simulink model "sixth_harmonic_concen"  (R2013a)
settings: Solver=ode4  StartTime=0.0  StopTime=0.1  FixedStep=Ts  RelTol=1e-3
values from neighbouring files (symbols this model uses):
  Cdc = 100e-6    (= 0.0001)    [acemp_sixth.m]    (also in immd_design_elen.m = 0.0002; immd_efficiency.m = 5e-05; immd_simulation_base.m = 5e-05; sixth_harmonic_report.m = 0.003)
  injfreq = 300*2*pi    (= 1884.95559215)    [acemp_sixth.m]
  injphase = k*pi/180    [acemp_sixth.m]
  injvoltmagn = 20    [acemp_sixth.m]
  Lload = Xload/wout_fund    [acemp_sixth.m]    (also in immd_base_varyingmod.m = Xload/wout; immd_design_elen.m = Xload/wout; immd_efficiency.m = Xload/wout; immd_simulation_base.m = Xload/wout)
  ma1 = 0.8    [acemp_sixth.m]
  ma3 = 0.5    [acemp_sixth.m]
  R1 = 5    [acemp_sixth.m]    (also in immd_efficiency.m; immd_simulation_base.m)
  Rload = Zload*pf    (= 17.306929152)    [acemp_sixth.m]    (also in immd_base_varyingmod.m = Zload*pf; immd_design_elen.m = Zload*pf; immd_efficiency.m = Zload*pf; immd_simulation_base.m = Zload*pf)
  Ts = 1e-6    (= 1e-06)    [acemp_sixth.m]    (also in immd_base_varyingmod.m = 1e-05; immd_design_elen.m; immd_efficiency.m; immd_simulation_base.m)
  V1 = Vdc*(R1+Rrefl)/Rrefl    (= 475.757575758)    [acemp_sixth.m]    (also in immd_efficiency.m = 526.262626263; immd_simulation_base.m = 425.252525253)
  wout_fund = 2*pi*fout_fund    (= 314.159265359)    [acemp_sixth.m]
  wout_three = 2*pi*fout_three    (= 942.477796077)    [acemp_sixth.m]
libraries: powerlib x33, powerlib_meascontrol x28
settings Model: Creator=ugurm  LastModifiedBy=ugurm

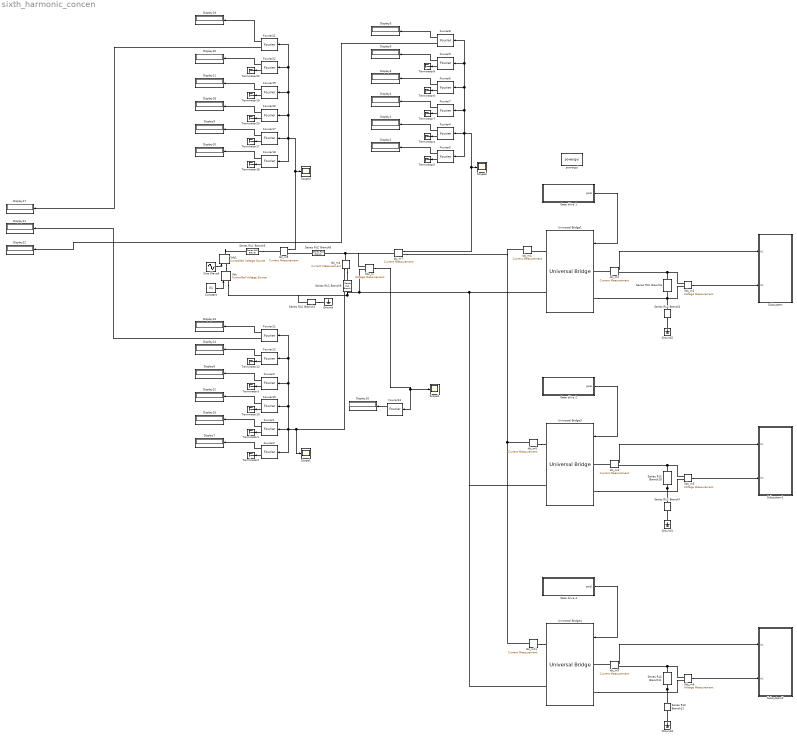
== system sixth_harmonic_concen ==
  Constant : Constant  Value=V1
  Display{1..22} (22 alike) : Display
  Fourier1 : powerlib_meascontrol/Measurements/Fourier  Freq=fout_fund  n=1  InInit=[0, 0]  Ts=Ts
  Fourier10 : powerlib_meascontrol/Measurements/Fourier  Freq=fout_fund  n=2  InInit=[0, 0]  Ts=Ts
  Fourier11 : powerlib_meascontrol/Measurements/Fourier  Freq=fout_fund  n=6  InInit=[0, 0]  Ts=Ts
  Fourier12 : powerlib_meascontrol/Measurements/Fourier  Freq=fout_fund  n=4  InInit=[0, 0]  Ts=Ts
  Fourier{2,5,13,18} (4 alike) : powerlib_meascontrol/Measurements/Fourier  Freq=fout_fund  n=0  InInit=[0, 0]  Ts=Ts
  Fourier17 : powerlib_meascontrol/Measurements/Fourier  Freq=fout_fund  n=1  InInit=[0, 0]  Ts=Ts
  Fourier19 : powerlib_meascontrol/Measurements/Fourier  Freq=fout_fund  n=3  InInit=[0, 0]  Ts=Ts
  Fourier20 : powerlib_meascontrol/Measurements/Fourier  Freq=fout_fund  n=2  InInit=[0, 0]  Ts=Ts
  Fourier21 : powerlib_meascontrol/Measurements/Fourier  Freq=fout_fund  n=6  InInit=[0, 0]  Ts=Ts
  Fourier22 : powerlib_meascontrol/Measurements/Fourier  Freq=fout_fund  n=4  InInit=[0, 0]  Ts=Ts
  Fourier3 : powerlib_meascontrol/Measurements/Fourier  Freq=fout_fund  n=3  InInit=[0, 0]  Ts=Ts
  Fourier4 : powerlib_meascontrol/Measurements/Fourier  Freq=fout_fund  n=1  InInit=[0, 0]  Ts=Ts
  Fourier6 : powerlib_meascontrol/Measurements/Fourier  Freq=fout_fund  n=3  InInit=[0, 0]  Ts=Ts
  Fourier7 : powerlib_meascontrol/Measurements/Fourier  Freq=fout_fund  n=2  InInit=[0, 0]  Ts=Ts
  Fourier8 : powerlib_meascontrol/Measurements/Fourier  Freq=fout_fund  n=6  InInit=[0, 0]  Ts=Ts
  Fourier9 : powerlib_meascontrol/Measurements/Fourier  Freq=fout_fund  n=4  InInit=[0, 0]  Ts=Ts
  Gate drive 1 : Subsystem
  Gate drive 2 : Subsystem
  Gate drive 4 : Subsystem
  Ground{,1..3} (4 alike) : powerlib/Elements/Ground  LConnTagsString=a
  Idc_m{1..7,9,11} (9 alike) : powerlib/Measurements/Current Measurement  PhasorSimulation=off  OutputType=Complex  PSBequivalent=0
  Scope{1..4} (4 alike) : Scope
      Scope1 settings: TimeRange=0.05  YMin=-15  YMax=42.5  SaveName=idc2
      Scope2 settings: TimeRange=0.05  YMin=380  YMax=422.5  SaveName=idc3
      Scope3 settings: TimeRange=0.05  YMin=-17.5  YMax=32.5  SaveName=idc
      Scope4 settings: TimeRange=0.05  YMin=10  YMax=25  SaveName=idc1
  Series RLC Branch10 : powerlib/Elements/Series RLC Branch  LConnTagsString=__new0  RConnTagsString=__new0  BranchType=RL  Resistance=Rload  Inductance=Lload  SetiL0=off  InitialCurrent=0  Capacitance=1e-6  Setx0=off  InitialVoltage=0  Measurements=None
  Series RLC Branch11 : powerlib/Elements/Series RLC Branch  LConnTagsString=__new0  RConnTagsString=__new0  BranchType=RL  Resistance=Rload  Inductance=Lload  SetiL0=off  InitialCurrent=0  Capacitance=1e-6  Setx0=off  InitialVoltage=0  Measurements=None
  Series RLC Branch{2..3,7,12} (4 alike) : powerlib/Elements/Series RLC Branch  LConnTagsString=__new0  RConnTagsString=__new0  BranchType=R  Resistance=1e12  Inductance=Lload  SetiL0=off  InitialCurrent=0  Capacitance=1e-6  Setx0=off  InitialVoltage=0  Measurements=None
  Series RLC Branch5 : powerlib/Elements/Series RLC Branch  LConnTagsString=__new0  RConnTagsString=__new0  BranchType=L  Resistance=1  Inductance=1e-3  SetiL0=off  InitialCurrent=0  Capacitance=1e-6  Setx0=off  InitialVoltage=0  Measurements=None
  Series RLC Branch6 : powerlib/Elements/Series RLC Branch  LConnTagsString=__new0  RConnTagsString=__new0  BranchType=RL  Resistance=Rload  Inductance=Lload  SetiL0=off  InitialCurrent=0  Capacitance=1e-6  Setx0=off  InitialVoltage=0  Measurements=None
  Series RLC Branch8 : powerlib/Elements/Series RLC Branch  LConnTagsString=__new0  RConnTagsString=__new0  BranchType=R  Resistance=R1  Inductance=Lload  SetiL0=off  InitialCurrent=0  Capacitance=1e-6  Setx0=off  InitialVoltage=0  Measurements=None
  Series RLC Branch9 : powerlib/Elements/Series RLC Branch  LConnTagsString=__new0  RConnTagsString=__new0  BranchType=C  Resistance=1e12  Inductance=Lload  SetiL0=off  InitialCurrent=0  Capacitance=Cdc  Setx0=off  InitialVoltage=0  Measurements=None
  Sine Wave3 : Sin  Amplitude=injvoltmagn  Frequency=injfreq  Phase=injphase  SampleTime=0
  Subsystem : Subsystem
  Subsystem1 : Subsystem
  Subsystem2 : Subsystem
  Terminator{1..7,9..10,12,17..20,22} (15 alike) : Terminator
  Universal Bridge1 : powerlib/Power Electronics/Universal Bridge  Arms=2  SnubberResistance=1e5  SnubberCapacitance=inf  Device=IGBT / Diodes  Ron=1e-6  Lon=0  ForwardVoltages="[  0  0  ]"  ForwardVoltage=0  GTOparameters=[ 10e-6 , 20e-6 ]  IGBTparameters=[0,0]  Measurements=None  Measurements_2=None  converterType=Rectifier
  Universal Bridge3 : powerlib/Power Electronics/Universal Bridge  Arms=2  SnubberResistance=1e5  SnubberCapacitance=inf  Device=IGBT / Diodes  Ron=1e-6  Lon=0  ForwardVoltages="[  0  0  ]"  ForwardVoltage=0  GTOparameters=[ 10e-6 , 20e-6 ]  IGBTparameters=[0,0]  Measurements=None  Measurements_2=None  converterType=Rectifier
  Universal Bridge4 : powerlib/Power Electronics/Universal Bridge  Arms=2  SnubberResistance=1e5  SnubberCapacitance=inf  Device=IGBT / Diodes  Ron=1e-6  Lon=0  ForwardVoltages="[  0  0  ]"  ForwardVoltage=0  GTOparameters=[ 10e-6 , 20e-6 ]  IGBTparameters=[0,0]  Measurements=None  Measurements_2=None  converterType=Rectifier
  Vdc : powerlib/Electrical Sources/Controlled Voltage Source  Initialize=off  Source_Type=DC  Amplitude=200  Phase=0  Frequency=0  Measurements=None
  Vdc1 : powerlib/Electrical Sources/Controlled Voltage Source  Initialize=off  Source_Type=DC  Amplitude=200  Phase=0  Frequency=0  Measurements=None
  Vdc_m{,2,5..6} (4 alike) : powerlib/Measurements/Voltage Measurement  PhasorSimulation=off  OutputType=Complex  PSBequivalent=0
  powergui : powerlib/powergui  Priority=1  SimulationMode=Discrete  SolverType=Tustin  SampleTime=Ts  frequency=60  SPID=off  DisableSnubberDevices=off  DisableRonSwitches=off  DisableVfSwitches=off  SwTol=0  Interpol=off  DisplayEquations=off  frequencyindice=0  Pbase=100e6  ErrMax=1e-4  Iterations=50  UnitsV=kV  UnitsW=MW  FunctionMessages=off  echomessages=off  HookPort=off  EnableUseOfTLC=off  x0status=blocks  RestoreLinks=warning  ResistiveCurrentMeasurement=off  Frange=[0:2:500]  Ylog=off  Xlog=on  ShowGrid=off  save=off  variable=ZData  structure=idc2  ZoomFFT=off  StartTime=0.02  cycles=4  DisplayStyle=2  fundamental=50  FreqAxis=off  MaxFrequency=1000  frequencyindicesteady=1  RmsSteady=1  display=off  Ts=0  methode=off
  wires:
  Gate drive 1/1(gate1) -> Universal Bridge1/1
  Fourier4/1 -> Display1/1
  Fourier4/2 -> Terminator4/1
  Fourier5/1 -> Display2/1
  Fourier5/2 -> Terminator5/1
  Fourier6/1 -> Display3/1
  Fourier6/2 -> Terminator6/1
  Fourier7/1 -> Display4/1
  Fourier7/2 -> Terminator7/1
  Fourier8/1 -> Display5/1
  Fourier8/2 -> Display22/1
  Idc_m7/1 -> Scope3/1, Fourier8/1, Fourier9/1, Fourier6/1, Fourier7/1, Fourier5/1, Fourier4/1
  Fourier9/1 -> Display6/1
  Fourier9/2 -> Terminator9/1
  Idc_m2/1 -> Subsystem/1(In1)
  Vdc_m2/1 -> Subsystem/2(In2)
  Gate drive 2/1(gate1) -> Universal Bridge3/1
  Idc_m3/1 -> Subsystem1/1(In1)
  Vdc_m5/1 -> Subsystem1/2(In2)
  Fourier17/1 -> Display9/1
  Fourier17/2 -> Terminator17/1
  Fourier18/1 -> Display10/1
  Fourier18/2 -> Terminator18/1
  Fourier19/1 -> Display11/1
  Fourier19/2 -> Terminator19/1
  Fourier20/1 -> Display18/1
  Fourier20/2 -> Terminator20/1
  Fourier21/1 -> Display19/1
  Fourier21/2 -> Display17/1
  Idc_m5/1 -> Scope4/1, Fourier21/1, Fourier22/1, Fourier19/1, Fourier20/1, Fourier18/1, Fourier17/1
  Fourier22/1 -> Display20/1
  Fourier22/2 -> Terminator22/1
  Gate drive 4/1(gate1) -> Universal Bridge4/1
  Idc_m9/1 -> Subsystem2/1(In1)
  Vdc_m6/1 -> Subsystem2/2(In2)
  Constant/1 -> Vdc/1
  Sine Wave3/1 -> Vdc1/1
  Fourier1/1 -> Display15/1
  Fourier1/2 -> Terminator1/1
  Fourier2/1 -> Display7/1
  Fourier2/2 -> Terminator2/1
  Fourier3/1 -> Display8/1
  Fourier3/2 -> Terminator3/1
  Fourier10/1 -> Display12/1
  Fourier10/2 -> Terminator10/1
  Fourier11/1 -> Display13/1
  Fourier11/2 -> Display21/1
  Idc_m4/1 -> Scope1/1, Fourier11/1, Fourier12/1, Fourier3/1, Fourier10/1, Fourier2/1, Fourier1/1
  Fourier12/1 -> Display14/1
  Fourier12/2 -> Terminator12/1
  Vdc_m/1 -> Fourier13/1, Scope2/1
  Fourier13/1 -> Display16/1
  connections:
  Universal Bridge1/RConn1 -- Idc_m1/RConn1
  Universal Bridge1/LConn2 -- Series RLC Branch2/LConn1 -- Vdc_m2/LConn2 -- Series RLC Branch6/RConn1
  Idc_m2/LConn1 -- Universal Bridge1/LConn1
  Series RLC Branch6/LConn1 -- Vdc_m2/LConn1 -- Idc_m2/RConn1
  Ground2/LConn1 -- Series RLC Branch2/RConn1
  Series RLC Branch9/RConn1 -- Vdc_m/LConn2 -- Universal Bridge1/RConn2 -- Universal Bridge4/RConn2 -- Universal Bridge3/RConn2 -- Vdc/LConn1 -- Series RLC Branch3/LConn1
  Idc_m4/LConn1 -- Vdc_m/LConn1 -- Idc_m7/LConn1 -- Series RLC Branch8/LConn1
  Series RLC Branch10/RConn1 -- Series RLC Branch7/LConn1 -- Universal Bridge3/LConn2 -- Vdc_m5/LConn2
  Series RLC Branch10/LConn1 -- Vdc_m5/LConn1 -- Idc_m3/RConn1
  Ground1/LConn1 -- Series RLC Branch7/RConn1
  Idc_m3/LConn1 -- Universal Bridge3/LConn1
  Idc_m6/RConn1 -- Universal Bridge3/RConn1
  Series RLC Branch11/RConn1 -- Series RLC Branch12/LConn1 -- Universal Bridge4/LConn2 -- Vdc_m6/LConn2
  Series RLC Branch11/LConn1 -- Vdc_m6/LConn1 -- Idc_m9/RConn1
  Ground3/LConn1 -- Series RLC Branch12/RConn1
  Idc_m9/LConn1 -- Universal Bridge4/LConn1
  Idc_m11/RConn1 -- Universal Bridge4/RConn1
  Series RLC Branch3/RConn1 -- Ground/LConn1
  Series RLC Branch8/RConn1 -- Idc_m5/RConn1
  Series RLC Branch5/LConn1 -- Idc_m5/LConn1
  Idc_m4/RConn1 -- Series RLC Branch9/LConn1
  Vdc1/RConn1 -- Series RLC Branch5/RConn1
  Vdc1/LConn1 -- Vdc/RConn1
  Idc_m11/LConn1 -- Idc_m1/LConn1 -- Idc_m7/RConn1 -- Idc_m6/LConn1

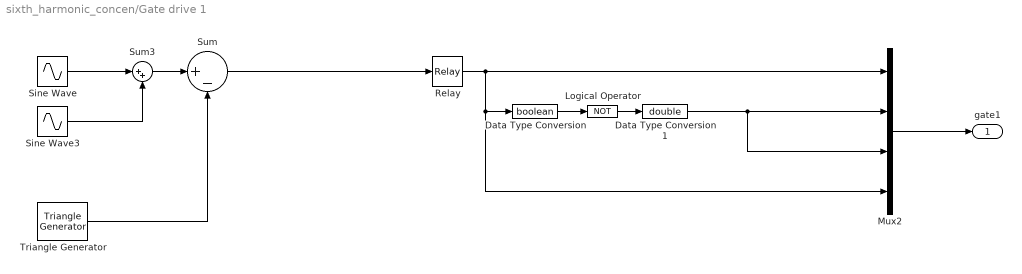
== system sixth_harmonic_concen/Gate drive 1 ==
  Data Type Conversion : DataTypeConversion  OutDataTypeStr=boolean
  Data Type Conversion1 : DataTypeConversion  OutDataTypeStr=double
  Logical Operator : Logic  Operator=NOT  AllPortsSameDT=off  OutDataTypeStr=boolean
  Mux2 : Mux
  Relay : Relay
  Sine Wave : Sin  Amplitude=ma1  Frequency=wout_fund  SampleTime=0
  Sine Wave3 : Sin  Amplitude=ma3  Frequency=wout_three  SampleTime=0
  Sum : Sum  Inputs=|+-
  Sum3 : Sum  Inputs=|++
  Triangle Generator : powerlib_meascontrol/Pulse & Signal Generators/Triangle Generator  Freq=fsw  Phase=0  Ts=Ts
  gate1 : Outport
  wires:
  Sum/1 -> Relay/1
  Data Type Conversion/1 -> Logical Operator/1
  Relay/1 -> Mux2/4, Data Type Conversion/1, Mux2/1
  Logical Operator/1 -> Data Type Conversion1/1
  Data Type Conversion1/1 -> Mux2/2, Mux2/3
  Mux2/1 -> gate1/1
  Sine Wave/1 -> Sum3/1
  Sine Wave3/1 -> Sum3/2
  Sum3/1 -> Sum/1
  Triangle Generator/1 -> Sum/2

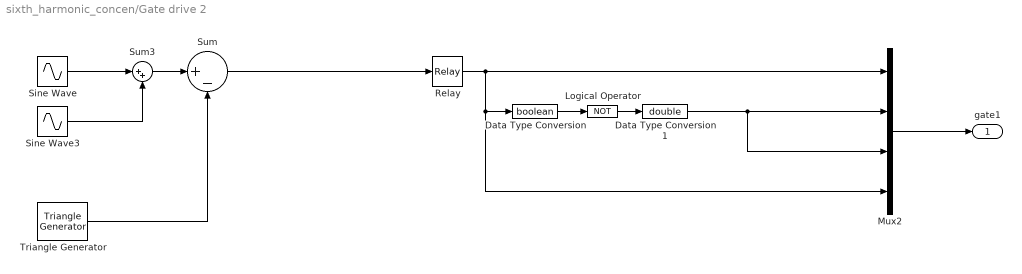
== system sixth_harmonic_concen/Gate drive 2 ==
  Data Type Conversion : DataTypeConversion  OutDataTypeStr=boolean
  Data Type Conversion1 : DataTypeConversion  OutDataTypeStr=double
  Logical Operator : Logic  Operator=NOT  AllPortsSameDT=off  OutDataTypeStr=boolean
  Mux2 : Mux
  Relay : Relay
  Sine Wave : Sin  Amplitude=ma1  Frequency=wout_fund  Phase=-2*pi/3  SampleTime=0
  Sine Wave3 : Sin  Amplitude=ma3  Frequency=wout_three  SampleTime=0
  Sum : Sum  Inputs=|+-
  Sum3 : Sum  Inputs=|++
  Triangle Generator : powerlib_meascontrol/Pulse & Signal Generators/Triangle Generator  Freq=fsw  Phase=0  Ts=Ts
  gate1 : Outport
  wires:
  Sum/1 -> Relay/1
  Data Type Conversion/1 -> Logical Operator/1
  Relay/1 -> Mux2/4, Data Type Conversion/1, Mux2/1
  Logical Operator/1 -> Data Type Conversion1/1
  Data Type Conversion1/1 -> Mux2/2, Mux2/3
  Mux2/1 -> gate1/1
  Sine Wave/1 -> Sum3/1
  Sine Wave3/1 -> Sum3/2
  Sum3/1 -> Sum/1
  Triangle Generator/1 -> Sum/2

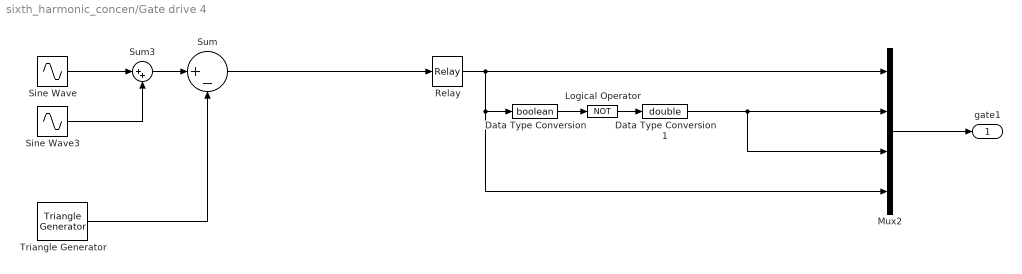
== system sixth_harmonic_concen/Gate drive 4 ==
  Data Type Conversion : DataTypeConversion  OutDataTypeStr=boolean
  Data Type Conversion1 : DataTypeConversion  OutDataTypeStr=double
  Logical Operator : Logic  Operator=NOT  AllPortsSameDT=off  OutDataTypeStr=boolean
  Mux2 : Mux
  Relay : Relay
  Sine Wave : Sin  Amplitude=ma1  Frequency=wout_fund  Phase=-4*pi/3  SampleTime=0
  Sine Wave3 : Sin  Amplitude=ma3  Frequency=wout_three  SampleTime=0
  Sum : Sum  Inputs=|+-
  Sum3 : Sum  Inputs=|++
  Triangle Generator : powerlib_meascontrol/Pulse & Signal Generators/Triangle Generator  Freq=fsw  Phase=0  Ts=Ts
  gate1 : Outport
  wires:
  Sum/1 -> Relay/1
  Data Type Conversion/1 -> Logical Operator/1
  Relay/1 -> Mux2/4, Data Type Conversion/1, Mux2/1
  Logical Operator/1 -> Data Type Conversion1/1
  Data Type Conversion1/1 -> Mux2/2, Mux2/3
  Mux2/1 -> gate1/1
  Sine Wave/1 -> Sum3/1
  Sine Wave3/1 -> Sum3/2
  Sum3/1 -> Sum/1
  Triangle Generator/1 -> Sum/2

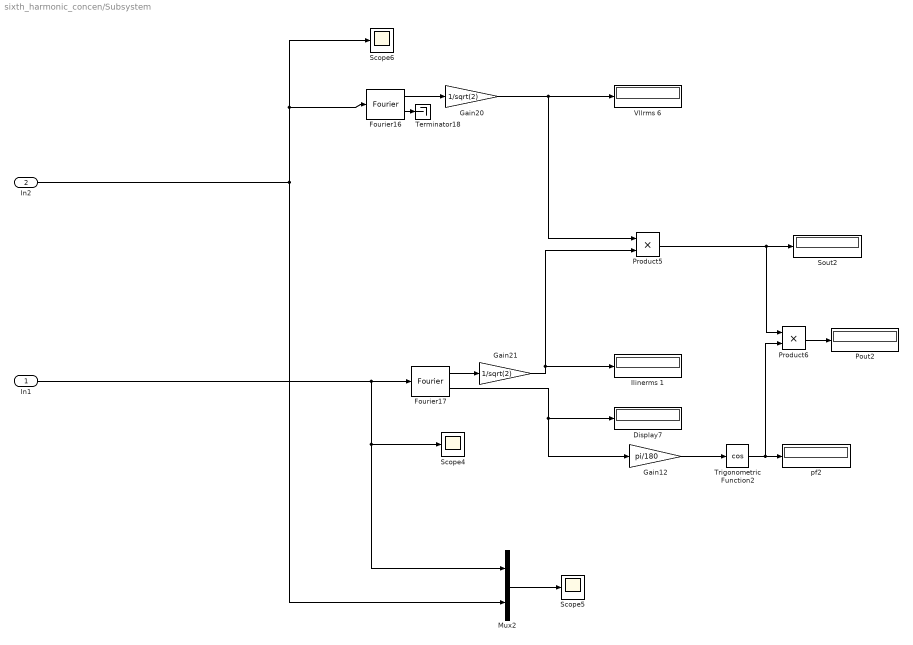
== system sixth_harmonic_concen/Subsystem ==
  In1 : Inport
  In2 : Inport  Port=2
  Display7 : Display
  Fourier16 : powerlib_meascontrol/Measurements/Fourier  Freq=fout_fund  n=1  InInit=[0, 0]  Ts=Ts
  Fourier17 : powerlib_meascontrol/Measurements/Fourier  Freq=fout_fund  n=1  InInit=[0, 0]  Ts=Ts
  Gain12 : Gain  Gain=pi/180
  Gain20 : Gain  Gain=1/sqrt(2)
  Gain21 : Gain  Gain=1/sqrt(2)
  Ilinerms 1 : Display
  Mux2 : Mux  Inputs=2
  Pout2 : Display
  Product5 : Product
  Product6 : Product
  Scope4 : Scope
      settings: YMin=32  YMax=45
  Scope5 : Scope
      settings: YMin=-700  YMax=700  SaveName=ScopeData2
  Scope6 : Scope
      settings: YMin=-400  YMax=400  SaveName=vline9
  Sout2 : Display
      settings: Format=short_e
  Terminator18 : Terminator
  Trigonometric Function2 : Trigonometry  Operator=cos
  Vllrms 6 : Display
  pf2 : Display
  wires:
  Mux2/1 -> Scope5/1
  In2/1 -> Scope6/1, Fourier16/1, Mux2/2
  In1/1 -> Fourier17/1, Scope4/1, Mux2/1
  Gain20/1 -> Product5/1, Vllrms 6/1
  Gain21/1 -> Ilinerms 1/1, Product5/2
  Fourier17/1 -> Gain21/1
  Trigonometric Function2/1 -> Product6/2, pf2/1
  Gain12/1 -> Trigonometric Function2/1
  Product6/1 -> Pout2/1
  Fourier16/1 -> Gain20/1
  Product5/1 -> Product6/1, Sout2/1
  Fourier17/2 -> Gain12/1, Display7/1
  Fourier16/2 -> Terminator18/1

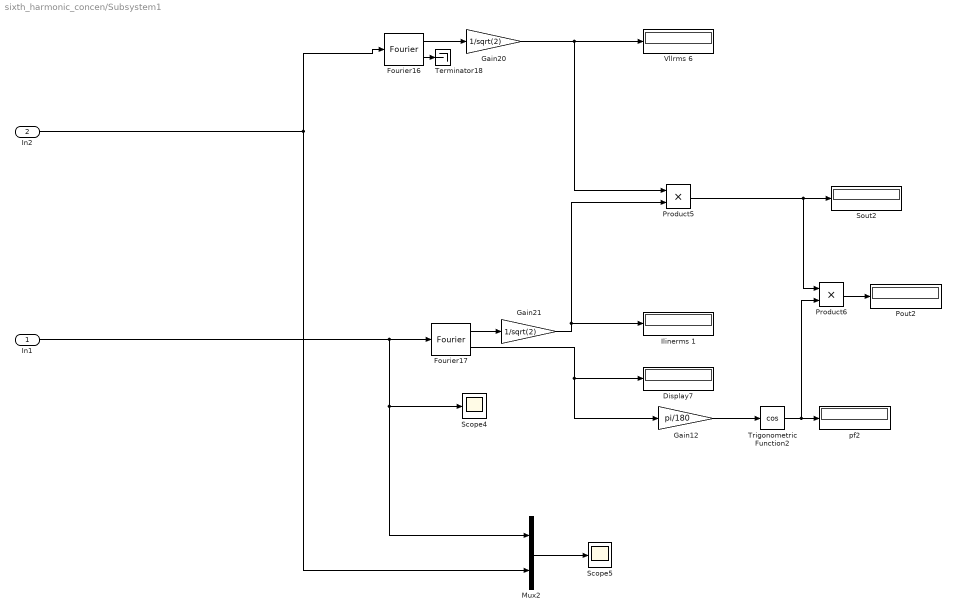
== system sixth_harmonic_concen/Subsystem1 ==
  In1 : Inport
  In2 : Inport  Port=2
  Display7 : Display
  Fourier16 : powerlib_meascontrol/Measurements/Fourier  Freq=fout_fund  n=1  InInit=[0, 0]  Ts=Ts
  Fourier17 : powerlib_meascontrol/Measurements/Fourier  Freq=fout_fund  n=1  InInit=[0, 0]  Ts=Ts
  Gain12 : Gain  Gain=pi/180
  Gain20 : Gain  Gain=1/sqrt(2)
  Gain21 : Gain  Gain=1/sqrt(2)
  Ilinerms 1 : Display
  Mux2 : Mux  Inputs=2
  Pout2 : Display
  Product5 : Product
  Product6 : Product
  Scope4 : Scope
      settings: YMin=32  YMax=45
  Scope5 : Scope
      settings: YMin=-700  YMax=700  SaveName=ScopeData2
  Sout2 : Display
      settings: Format=short_e
  Terminator18 : Terminator
  Trigonometric Function2 : Trigonometry  Operator=cos
  Vllrms 6 : Display
  pf2 : Display
  wires:
  Mux2/1 -> Scope5/1
  In2/1 -> Fourier16/1, Mux2/2
  In1/1 -> Fourier17/1, Scope4/1, Mux2/1
  Gain20/1 -> Product5/1, Vllrms 6/1
  Gain21/1 -> Ilinerms 1/1, Product5/2
  Fourier17/1 -> Gain21/1
  Trigonometric Function2/1 -> Product6/2, pf2/1
  Gain12/1 -> Trigonometric Function2/1
  Product6/1 -> Pout2/1
  Fourier16/1 -> Gain20/1
  Product5/1 -> Product6/1, Sout2/1
  Fourier17/2 -> Gain12/1, Display7/1
  Fourier16/2 -> Terminator18/1

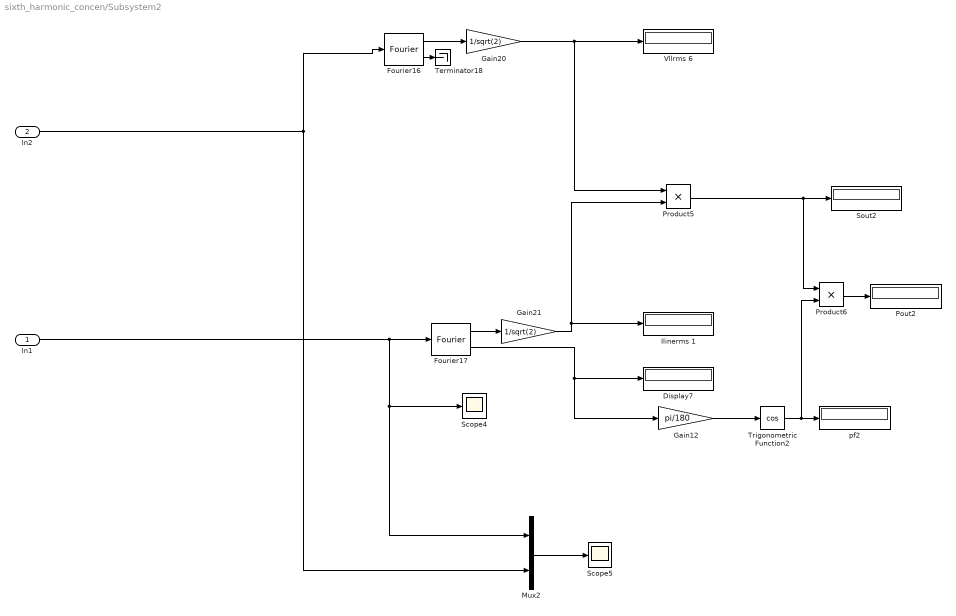
== system sixth_harmonic_concen/Subsystem2 ==
  In1 : Inport
  In2 : Inport  Port=2
  Display7 : Display
  Fourier16 : powerlib_meascontrol/Measurements/Fourier  Freq=fout_fund  n=1  InInit=[0, 0]  Ts=Ts
  Fourier17 : powerlib_meascontrol/Measurements/Fourier  Freq=fout_fund  n=1  InInit=[0, 0]  Ts=Ts
  Gain12 : Gain  Gain=pi/180
  Gain20 : Gain  Gain=1/sqrt(2)
  Gain21 : Gain  Gain=1/sqrt(2)
  Ilinerms 1 : Display
  Mux2 : Mux  Inputs=2
  Pout2 : Display
  Product5 : Product
  Product6 : Product
  Scope4 : Scope
      settings: YMin=32  YMax=45
  Scope5 : Scope
      settings: YMin=-700  YMax=700  SaveName=ScopeData2
  Sout2 : Display
      settings: Format=short_e
  Terminator18 : Terminator
  Trigonometric Function2 : Trigonometry  Operator=cos
  Vllrms 6 : Display
  pf2 : Display
  wires:
  Mux2/1 -> Scope5/1
  In2/1 -> Fourier16/1, Mux2/2
  In1/1 -> Fourier17/1, Scope4/1, Mux2/1
  Gain20/1 -> Product5/1, Vllrms 6/1
  Gain21/1 -> Ilinerms 1/1, Product5/2
  Fourier17/1 -> Gain21/1
  Trigonometric Function2/1 -> Product6/2, pf2/1
  Gain12/1 -> Trigonometric Function2/1
  Product6/1 -> Pout2/1
  Fourier16/1 -> Gain20/1
  Product5/1 -> Product6/1, Sout2/1
  Fourier17/2 -> Gain12/1, Display7/1
  Fourier16/2 -> Terminator18/1
